simulink model "quadrotorModel"  (R2022a)
settings: Solver=VariableStepAuto  StartTime=0.0  StopTime=10.0  RelTol=1e-3
model workspace (MAT data in the model file):
  x0 = 0
settings Model: Creator=zheyu  LastModifiedBy=zheyu

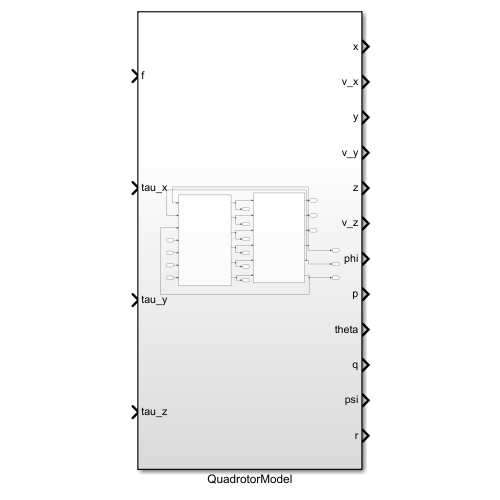
[thumbnail: Simulink's stored preview of the top-level diagram]
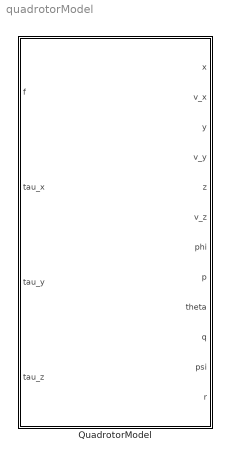
== system quadrotorModel ==
  QuadrotorModel : Subsystem

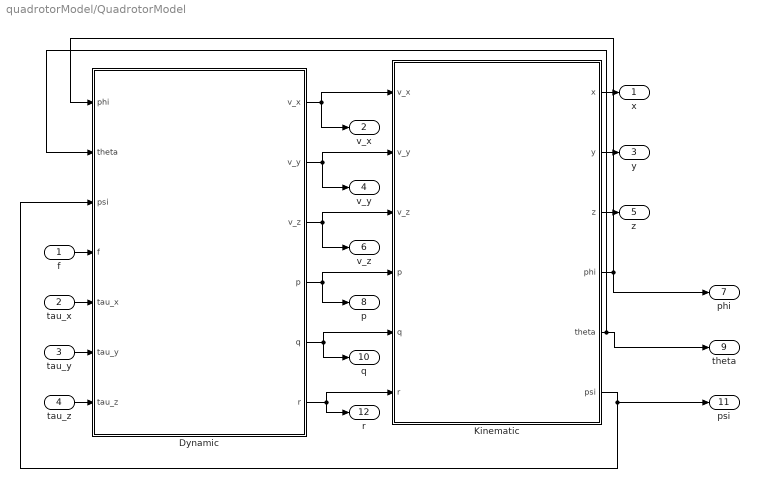
== system quadrotorModel/QuadrotorModel ==
  f : Inport
  tau_x : Inport  Port=2
  tau_y : Inport  Port=3
  tau_z : Inport  Port=4
  Dynamic : Subsystem
  Kinematic : Subsystem
  x : Outport
  v_x : Outport  Port=2
  y : Outport  Port=3
  v_y : Outport  Port=4
  z : Outport  Port=5
  v_z : Outport  Port=6
  phi : Outport  Port=7
  p : Outport  Port=8
  theta : Outport  Port=9
  q : Outport  Port=10
  psi : Outport  Port=11
  r : Outport  Port=12
  wires:
  Dynamic/3(v_z) -> Kinematic/3(v_z), v_z/1
  Dynamic/6(r) -> Kinematic/6(r), r/1
  tau_y/1 -> Dynamic/6(tau_y)
  Dynamic/2(v_y) -> Kinematic/2(v_y), v_y/1
  Dynamic/5(q) -> Kinematic/5(q), q/1
  Dynamic/4(p) -> Kinematic/4(p), p/1
  Kinematic/3(z) -> z/1
  Kinematic/6(psi) -> psi/1, Dynamic/3(psi)
  tau_z/1 -> Dynamic/7(tau_z)
  Dynamic/1(v_x) -> Kinematic/1(v_x), v_x/1
  Kinematic/4(phi) -> phi/1, Dynamic/1(phi)
  Kinematic/5(theta) -> theta/1, Dynamic/2(theta)
  f/1 -> Dynamic/4(f)
  tau_x/1 -> Dynamic/5(tau_x)
  Kinematic/2(y) -> y/1
  Kinematic/1(x) -> x/1

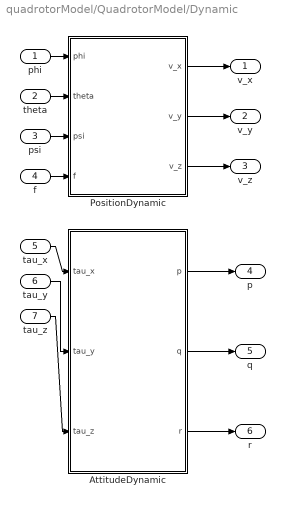
== system quadrotorModel/QuadrotorModel/Dynamic ==
  phi : Inport
  theta : Inport  Port=2
  psi : Inport  Port=3
  f : Inport  Port=4
  tau_x : Inport  Port=5
  tau_y : Inport  Port=6
  tau_z : Inport  Port=7
  AttitudeDynamic : Subsystem
  PositionDynamic : Subsystem
  v_x : Outport
  v_y : Outport  Port=2
  v_z : Outport  Port=3
  p : Outport  Port=4
  q : Outport  Port=5
  r : Outport  Port=6
  wires:
  phi/1 -> PositionDynamic/1(phi)
  tau_x/1 -> AttitudeDynamic/1(tau_x)
  AttitudeDynamic/1(p) -> p/1
  PositionDynamic/2(v_y) -> v_y/1
  theta/1 -> PositionDynamic/2(theta)
  tau_y/1 -> AttitudeDynamic/2(tau_y)
  AttitudeDynamic/2(q) -> q/1
  f/1 -> PositionDynamic/4(f)
  psi/1 -> PositionDynamic/3(psi)
  tau_z/1 -> AttitudeDynamic/3(tau_z)
  PositionDynamic/1(v_x) -> v_x/1
  AttitudeDynamic/3(r) -> r/1
  PositionDynamic/3(v_z) -> v_z/1

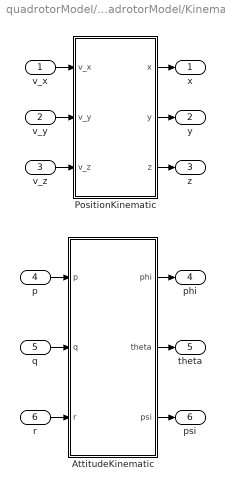
== system quadrotorModel/QuadrotorModel/Kinematic ==
  v_x : Inport
  v_y : Inport  Port=2
  v_z : Inport  Port=3
  p : Inport  Port=4
  q : Inport  Port=5
  r : Inport  Port=6
  AttitudeKinematic : Subsystem
  PositionKinematic : Subsystem
  x : Outport
  y : Outport  Port=2
  z : Outport  Port=3
  phi : Outport  Port=4
  theta : Outport  Port=5
  psi : Outport  Port=6
  wires:
  p/1 -> AttitudeKinematic/1(p)
  v_x/1 -> PositionKinematic/1(v_x)
  PositionKinematic/2(y) -> y/1
  PositionKinematic/3(z) -> z/1
  PositionKinematic/1(x) -> x/1
  AttitudeKinematic/1(phi) -> phi/1
  q/1 -> AttitudeKinematic/2(q)
  v_y/1 -> PositionKinematic/2(v_y)
  v_z/1 -> PositionKinematic/3(v_z)
  r/1 -> AttitudeKinematic/3(r)
  AttitudeKinematic/3(psi) -> psi/1
  AttitudeKinematic/2(theta) -> theta/1

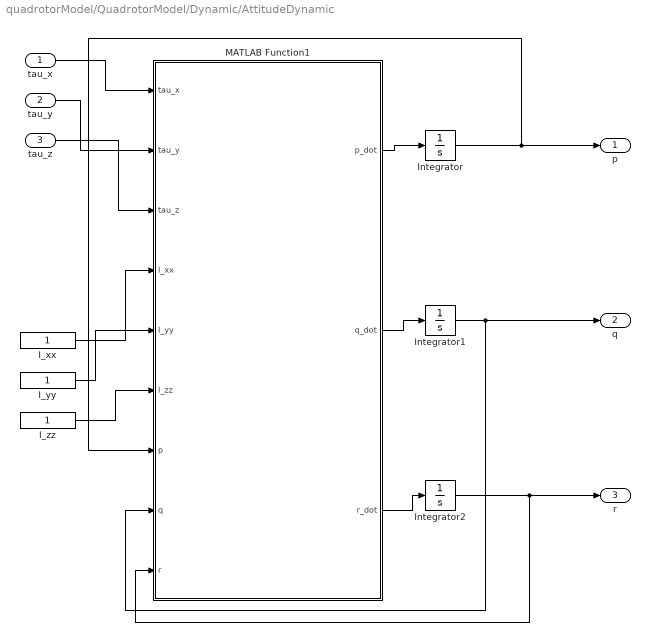
== system quadrotorModel/QuadrotorModel/Dynamic/AttitudeDynamic ==
  tau_x : Inport
  tau_y : Inport  Port=2
  tau_z : Inport  Port=3
  I_xx : Constant
  I_yy : Constant
  I_zz : Constant
  Integrator : Integrator
  Integrator1 : Integrator
  Integrator2 : Integrator
  MATLAB Function1 : MATLAB Function  TreatAsAtomicUnit=on
  p : Outport
  q : Outport  Port=2
  r : Outport  Port=3
  wires:
  I_yy/1 -> MATLAB Function1/5(I_yy)
  Integrator/1 -> p/1, MATLAB Function1/7(p)
  I_zz/1 -> MATLAB Function1/6(I_zz)
  MATLAB Function1/2(q_dot) -> Integrator1/1
  Integrator1/1 -> q/1, MATLAB Function1/8(q)
  Integrator2/1 -> r/1, MATLAB Function1/9(r)
  MATLAB Function1/1(p_dot) -> Integrator/1
  MATLAB Function1/3(r_dot) -> Integrator2/1
  I_xx/1 -> MATLAB Function1/4(I_xx)
  tau_z/1 -> MATLAB Function1/3(tau_z)
  tau_y/1 -> MATLAB Function1/2(tau_y)
  tau_x/1 -> MATLAB Function1/1(tau_x)

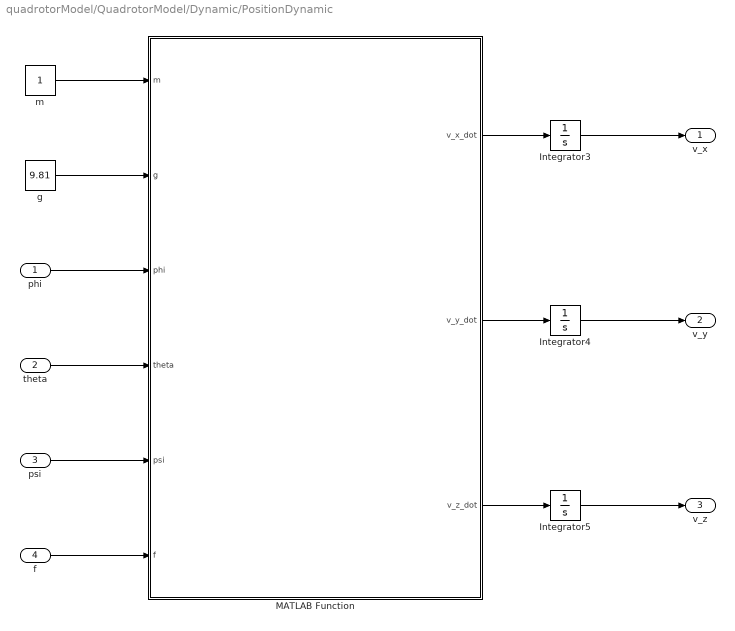
== system quadrotorModel/QuadrotorModel/Dynamic/PositionDynamic ==
  phi : Inport
  theta : Inport  Port=2
  psi : Inport  Port=3
  f : Inport  Port=4
  Integrator3 : Integrator
  Integrator4 : Integrator
  Integrator5 : Integrator
  MATLAB Function : MATLAB Function  TreatAsAtomicUnit=on
  g : Constant  Value=9.81
  m : Constant
  v_x : Outport
  v_y : Outport  Port=2
  v_z : Outport  Port=3
  wires:
  Integrator5/1 -> v_z/1
  MATLAB Function/2(v_y_dot) -> Integrator4/1
  MATLAB Function/3(v_z_dot) -> Integrator5/1
  psi/1 -> MATLAB Function/5(psi)
  MATLAB Function/1(v_x_dot) -> Integrator3/1
  g/1 -> MATLAB Function/2(g)
  theta/1 -> MATLAB Function/4(theta)
  Integrator3/1 -> v_x/1
  m/1 -> MATLAB Function/1(m)
  f/1 -> MATLAB Function/6(f)
  phi/1 -> MATLAB Function/3(phi)
  Integrator4/1 -> v_y/1

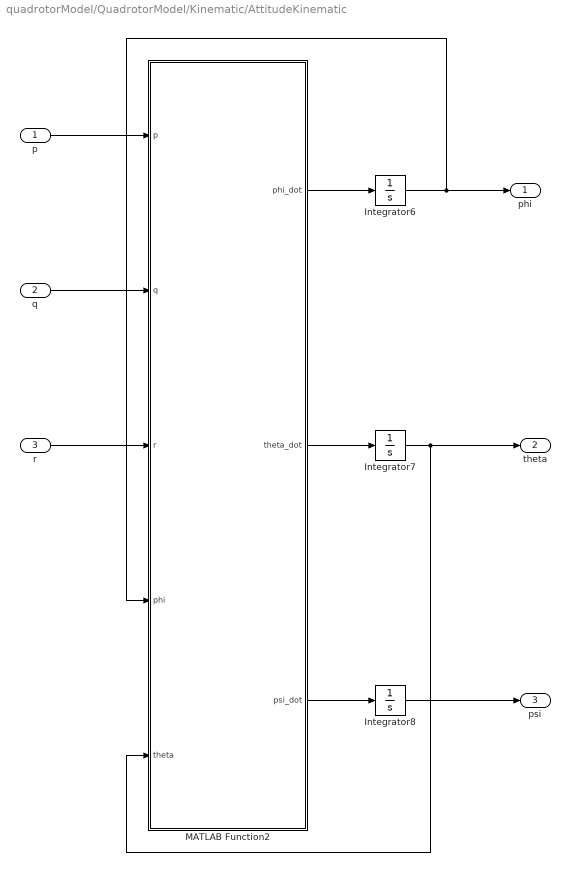
== system quadrotorModel/QuadrotorModel/Kinematic/AttitudeKinematic ==
  p : Inport
  q : Inport  Port=2
  r : Inport  Port=3
  Integrator6 : Integrator
  Integrator7 : Integrator
  Integrator8 : Integrator
  MATLAB Function2 : MATLAB Function  TreatAsAtomicUnit=on
  phi : Outport
  theta : Outport  Port=2
  psi : Outport  Port=3
  wires:
  r/1 -> MATLAB Function2/3(r)
  MATLAB Function2/1(phi_dot) -> Integrator6/1
  Integrator8/1 -> psi/1
  MATLAB Function2/3(psi_dot) -> Integrator8/1
  MATLAB Function2/2(theta_dot) -> Integrator7/1
  Integrator6/1 -> phi/1, MATLAB Function2/4(phi)
  Integrator7/1 -> theta/1, MATLAB Function2/5(theta)
  q/1 -> MATLAB Function2/2(q)
  p/1 -> MATLAB Function2/1(p)

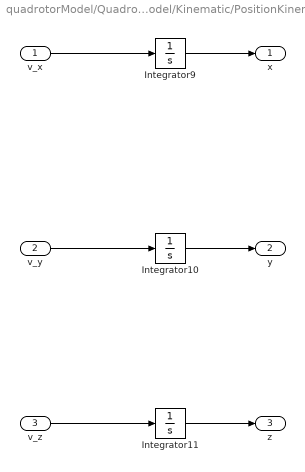
== system quadrotorModel/QuadrotorModel/Kinematic/PositionKinematic ==
  v_x : Inport
  v_y : Inport  Port=2
  v_z : Inport  Port=3
  Integrator10 : Integrator
  Integrator11 : Integrator
  Integrator9 : Integrator
  x : Outport
  y : Outport  Port=2
  z : Outport  Port=3
  wires:
  v_x/1 -> Integrator9/1
  v_y/1 -> Integrator10/1
  Integrator10/1 -> y/1
  Integrator11/1 -> z/1
  v_z/1 -> Integrator11/1
  Integrator9/1 -> x/1

== matlab function quadrotorModel/QuadrotorModel/Dynamic/AttitudeDynamic/MATLAB Function1 ==
  data: tau_x input; p_dot output; tau_y input; tau_z input; I_xx input; I_yy input; I_zz input; p input; q input; r input; q_dot output; r_dot output
function [p_dot, q_dot, r_dot] = AttitudeDynamic(tau_x, tau_y, tau_z, I_xx, I_yy, I_zz, p,q,r)

p_dot = (1/I_xx) * (tau_x + q *r * (I_yy-I_zz));
q_dot = (1/I_yy) * (tau_y + p *r * (I_zz-I_xx));
r_dot = (1/I_zz) * (tau_z + p *q * (I_xx-I_yy));

end

== matlab function quadrotorModel/QuadrotorModel/Dynamic/PositionDynamic/MATLAB Function ==
  data: m input; v_x_dot output; v_y_dot output; g input; phi input; theta input; psi input; f input; v_z_dot output
function [v_x_dot, v_y_dot, v_z_dot] = PositionDynamic(m, g, phi, theta, psi, f)

v_x_dot = -f * (1/m) * (cos(psi) * sin(theta) * cos(phi) + sin(psi) * sin(phi));
v_y_dot = -f * (1/m) * (sin(psi) * sin(theta) * cos(phi) - cos(psi) * sin(phi));
v_z_dot = g - f * (1/m) * cos(phi) * cos(theta);
end

== matlab function quadrotorModel/QuadrotorModel/Kinematic/AttitudeKinematic/MATLAB Function2 ==
  data: p input; phi_dot output; q input; r input; phi input; theta input; theta_dot output; psi_dot output
function [phi_dot, theta_dot, psi_dot] = AttitudeKinematic(p, q, r, phi, theta)

phi_dot = p + q *tan(theta) * sin(phi) + r * tan(theta) * cos(phi);
theta_dot = q * cos(phi) - r * sin(phi);
psi_dot = (q * sin(phi) + r *cos(phi) / cos(theta));

end
